simulink model "Week2_Problem2"  (R2020b)
settings: Solver=VariableStepAuto  StartTime=0.0  StopTime=10.0  RelTol=1e-3
values from neighbouring files (symbols this model uses):
  be = 2.0    [Problem2_data.sldd]
  bv = 1.0    [Problem2_data.sldd]
  Fn : value not decoded    [Problem2_data.sldd]
  le = 1.0    [Problem2_data.sldd]
  lv = 5.0    [Problem2_data.sldd]
  muk = 1.0    [Problem2_data.sldd]
  mus = 1.5    [Problem2_data.sldd]
  R = 1.0    [Problem2_data.sldd]
  Tin : value not decoded    [Problem2_data.sldd]
undefined symbols (not defined in the file or in its folder): v
settings Model: Creator=ASUS  LastModifiedBy=ASUS

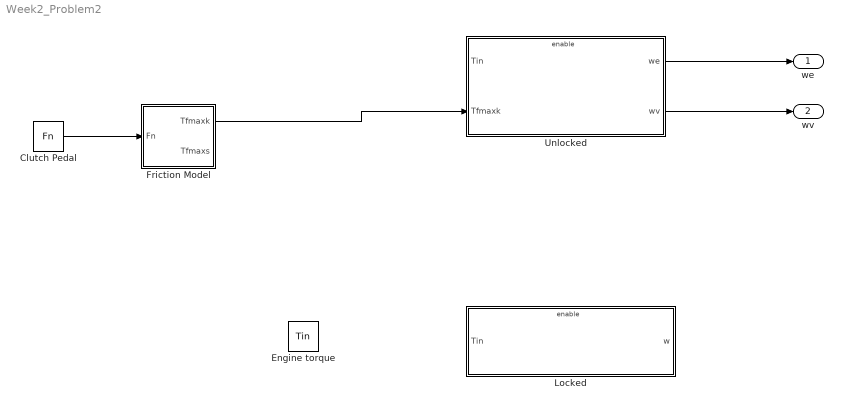
== system Week2_Problem2 ==
  Clutch Pedal : Constant  Value=Fn
  Engine torque : Constant  Value=Tin
  Friction Model : Subsystem
  Locked : Subsystem
  Unlocked : Subsystem
  we : Outport
  wv : Outport  Port=2
  wires:
  Clutch Pedal/1 -> Friction Model/1(Fn)
  Friction Model/1(Tfmaxk) -> Unlocked/2(Tfmaxk)
  Unlocked/1(we) -> we/1
  Unlocked/2(wv) -> wv/1

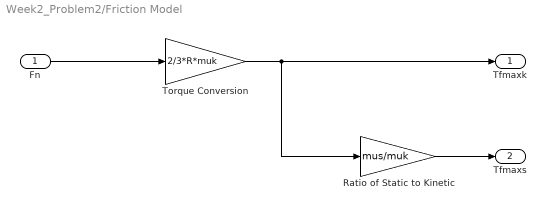
== system Week2_Problem2/Friction Model ==
  Fn : Inport
  Ratio of Static to Kinetic : Gain  Gain=mus/muk
  Torque Conversion : Gain  Gain=2/3*R*muk
  Tfmaxk : Outport
  Tfmaxs : Outport  Port=2
  wires:
  Ratio of Static to Kinetic/1 -> Tfmaxs/1
  Torque Conversion/1 -> Tfmaxk/1, Ratio of Static to Kinetic/1
  Fn/1 -> Torque Conversion/1

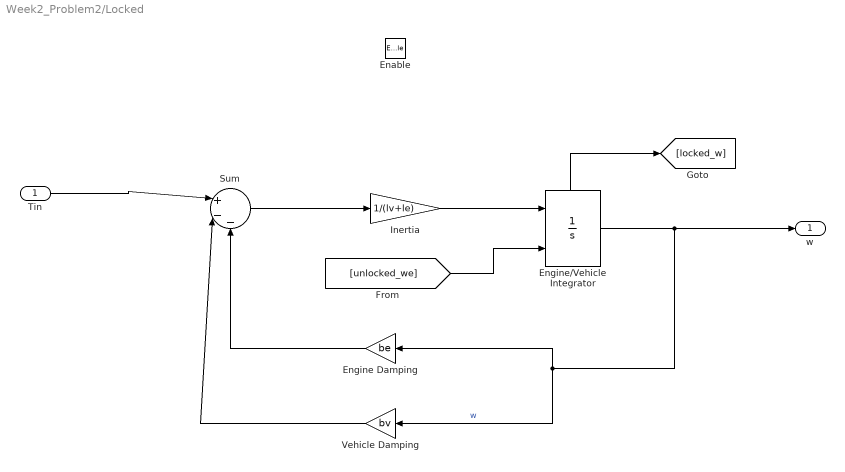
== system Week2_Problem2/Locked ==
  Tin : Inport
  Enable : EnablePort
  Engine Damping : Gain  Gain=be
  Engine/Vehicle Integrator : Integrator  InitialConditionSource=external  ShowStatePort=on
  Inertia : Gain  Gain=1/(lv+le)
  Sum : Sum  Inputs=|+--
  Vehicle Damping : Gain  Gain=bv
  w : Outport
  wires:
  Engine/Vehicle Integrator/1 -> w/1, Engine Damping/1, Vehicle Damping/1  "w"
  [unlocked_we] -> Engine/Vehicle Integrator/2
  Tin/1 -> Sum/1
  Inertia/1 -> Engine/Vehicle Integrator/1
  Sum/1 -> Inertia/1
  Engine/Vehicle Integrator/State -> [locked_w]
  Engine Damping/1 -> Sum/3
  Vehicle Damping/1 -> Sum/2

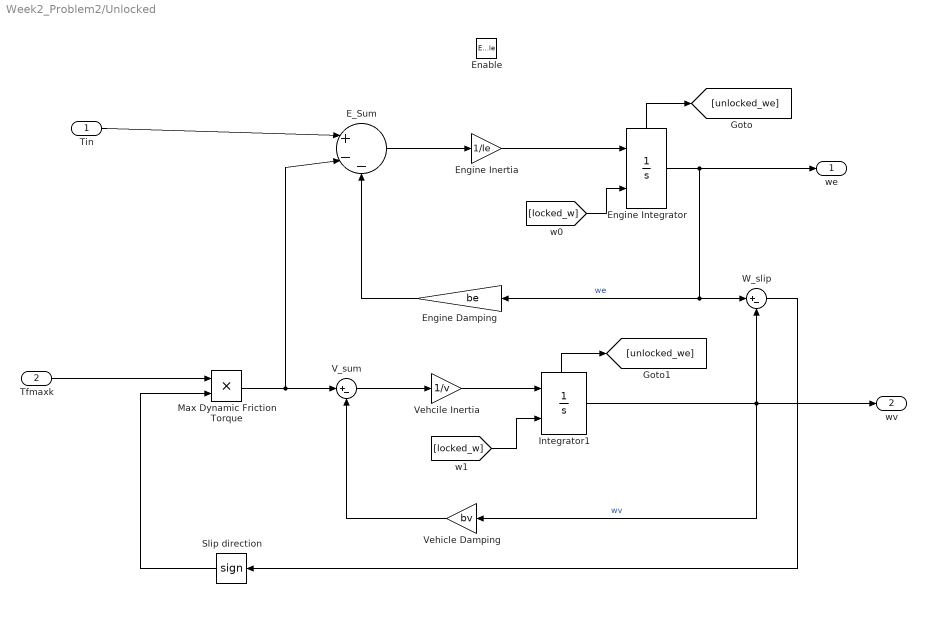
== system Week2_Problem2/Unlocked ==
  Tin : Inport
  Tfmaxk : Inport  Port=2
  Enable : EnablePort
  E_Sum : Sum  Inputs=|+--
  Engine Damping : Gain  Gain=be
  Engine Inertia : Gain  Gain=1/le
  Engine Integrator : Integrator  InitialConditionSource=external  ShowStatePort=on
  Integrator1 : Integrator  InitialConditionSource=external  ShowStatePort=on
  Max Dynamic Friction Torque : Product
  Slip direction : Signum
  V_sum : Sum  Inputs=|+-
  Vehcile Inertia : Gain  Gain=1/v
  Vehicle Damping : Gain  Gain=bv
  W_slip : Sum  Inputs=|+-
  we : Outport
  wv : Outport  Port=2
  wires:
  Integrator1/State -> [unlocked_we]
  Engine Inertia/1 -> Engine Integrator/1
  Max Dynamic Friction Torque/1 -> E_Sum/2, V_sum/1
  Engine Integrator/1 -> we/1, W_slip/1, Engine Damping/1  "we"
  Vehicle Damping/1 -> V_sum/2
  Slip direction/1 -> Max Dynamic Friction Torque/2
  V_sum/1 -> Vehcile Inertia/1
  Integrator1/1 -> wv/1, Vehicle Damping/1, W_slip/2  "wv"
  Tfmaxk/1 -> Max Dynamic Friction Torque/1
  Vehcile Inertia/1 -> Integrator1/1
  [locked_w] -> Integrator1/2
  [locked_w] -> Engine Integrator/2
  Engine Integrator/State -> [unlocked_we]
  E_Sum/1 -> Engine Inertia/1
  Engine Damping/1 -> E_Sum/3
  W_slip/1 -> Slip direction/1
  Tin/1 -> E_Sum/1
